simulink model "simulink_lqr"  (R2022b)
settings: Solver=ode15s  StartTime=0.0  StopTime=1  RelTol=1e-3
values from neighbouring files (symbols this model uses):
  x0 = xLp + [x,y,z, zeros(1,9)]'    [convergence_plot_func.m]
undefined symbols (not defined in the file or in its folder): Kred, params, uLp, xLp
settings Model: Creator=pal12  LastModifiedBy=pal12

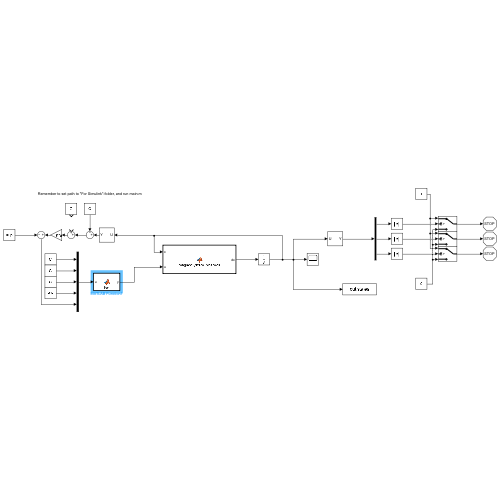
[thumbnail: Simulink's stored preview of the top-level diagram]
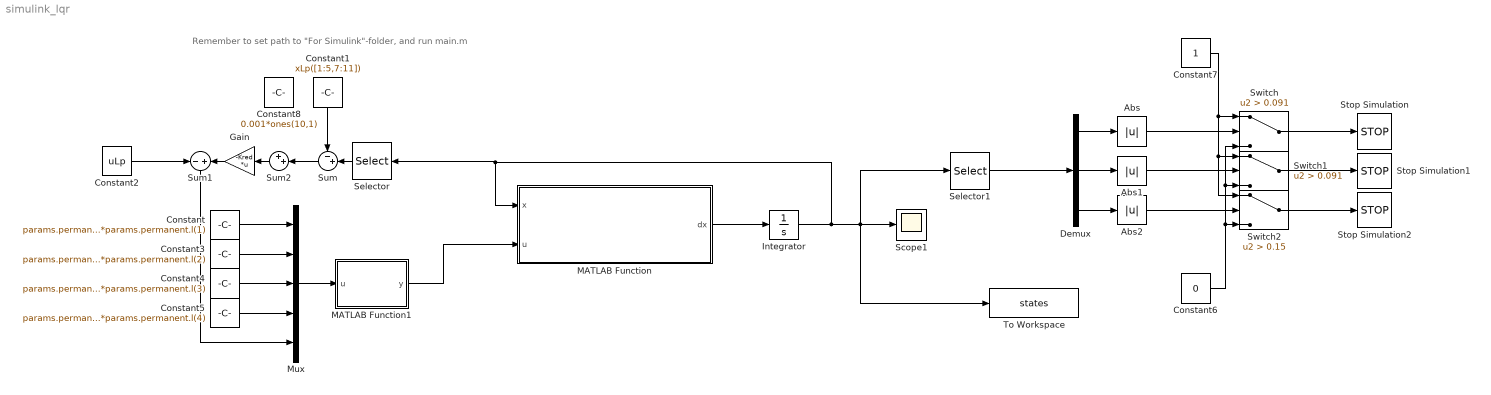
== system simulink_lqr ==
  note: Remember to set path to "For Simulink"-folder, and run main.m
  Abs : Abs  SaturateOnIntegerOverflow=off
  Abs1 : Abs  SaturateOnIntegerOverflow=off
  Abs2 : Abs  SaturateOnIntegerOverflow=off
  Constant : Constant  Value=params.permanent.J/params.physical.mu0*params.permanent.l(1)
  Constant1 : Constant  Value=xLp([1:5,7:11])
  Constant2 : Constant  Value=uLp
  Constant3 : Constant  Value=params.permanent.J/params.physical.mu0*params.permanent.l(2)
  Constant4 : Constant  Value=params.permanent.J/params.physical.mu0*params.permanent.l(3)
  Constant5 : Constant  Value=params.permanent.J/params.physical.mu0*params.permanent.l(4)
  Constant6 : Constant  Value=0
  Constant7 : Constant
  Constant8 : Constant  Value=0.001*ones(10,1)
  Demux : Demux  Outputs=3
  Gain : Gain  Gain=-Kred  Multiplication=Matrix(K*u)
  Integrator : Integrator  InitialCondition=x0
  MATLAB Function : MATLAB Function  TreatAsAtomicUnit=on
  MATLAB Function1 : MATLAB Function  TreatAsAtomicUnit=on
  Mux : Mux  Inputs=5
  Scope1 : Scope
  Selector : Selector  InputPortWidth=12  IndexOptions=Index vector (dialog)  Indices=[1 2 3 4 5 7 8 9 10 11]  OutputSizes=1
  Selector1 : Selector  InputPortWidth=12  IndexOptions=Index vector (dialog)  Indices=[1 2 3]  OutputSizes=1
  Stop Simulation : Stop
  Stop Simulation1 : Stop
  Stop Simulation2 : Stop
  Sum : Sum  Inputs=-+|
  Sum1 : Sum  Inputs=-|+
  Sum2 : Sum  Inputs=++|
  Switch : Switch  Criteria=u2 > Threshold  Threshold=0.091  SaturateOnIntegerOverflow=off  InputSameDT=off
  Switch1 : Switch  Criteria=u2 > Threshold  Threshold=0.091  SaturateOnIntegerOverflow=off  InputSameDT=off
  Switch2 : Switch  Criteria=u2 > Threshold  Threshold=0.15  SaturateOnIntegerOverflow=off  InputSameDT=off
  To Workspace : ToWorkspace  VariableName=states  SampleTime=-1
  wires:
  MATLAB Function/1(dx) -> Integrator/1
  Constant1/1 -> Sum/1
  Gain/1 -> Sum1/2
  Constant2/1 -> Sum1/1
  Sum1/1 -> Mux/5
  Constant/1 -> Mux/1
  Constant3/1 -> Mux/2
  Constant4/1 -> Mux/3
  Constant5/1 -> Mux/4
  Selector/1 -> Sum/2
  Selector1/1 -> Demux/1
  Demux/1 -> Abs/1
  Demux/2 -> Abs1/1
  Demux/3 -> Abs2/1
  Abs2/1 -> Switch2/2
  Abs1/1 -> Switch1/2
  Abs/1 -> Switch/2
  Constant6/1 -> Switch/3, Switch1/3, Switch2/3
  Constant7/1 -> Switch/1, Switch2/1, Switch1/1
  Switch/1 -> Stop Simulation/1
  Switch1/1 -> Stop Simulation1/1
  Switch2/1 -> Stop Simulation2/1
  Sum2/1 -> Gain/1
  Sum/1 -> Sum2/2
  Mux/1 -> MATLAB Function1/1(u)
  Integrator/1 -> Selector/1, MATLAB Function/1(x), Scope1/1, Selector1/1, To Workspace/1
  MATLAB Function1/1(y) -> MATLAB Function/2(u)

== matlab function simulink_lqr/MATLAB Function1 ==
  data: u input; y output
function y = fcn(u)
lim = 150;
for i=1:4
    if u(i) < -lim
        u(i) = -lim;
    elseif u(i) > lim
        u(i) = lim;
    end
end
y = u;

== matlab function simulink_lqr/MATLAB Function ==
  data: x input; u input; dx output; params parameter
function dx = maglevSystemDynamics(x,u,params)
    %{
    Computes the derivative of the state for a magnetic levitation system.
    - x: current state
    - u: control input
    - params: system parameters
    %}

    % Computing force and torque on levitating magnet
    [Fm,Fs,taum,taus] = computeForceAndTorque(x,0,params,"fast");

    F = Fm*u(1:4)+Fs*u(5:8);
    tau = taum*u(1:4)+taus*u(5:8);
    
    % Setting up system matrices
    A = [
        zeros(6), eye(6);
        zeros(6), zeros(6)
        ];

    B = [
        zeros(6);
        eye(6)
        ];
    
    % Mass and inertia properties of the magnet
    M = [
        params.magnet.m*eye(3), zeros(3);
        zeros(3), diag(params.magnet.I)
        ];
    
    % Computing the nonlinear function f(x,u)
    f = M\([F;tau]-[zeros(3,1); cross(x(10:12),diag(params.magnet.I)*x(10:12))])-[zeros(2,1);params.physical.g;zeros(3,1)];
    
    dx = A*x+B*f;
end
